simulink model "simplificado"  (R2016a)
settings: Solver=VariableStepAuto  StartTime=0.0  StopTime=10.0  RelTol=1e-3
undefined symbols (not defined in the file or in its folder): h, K1, K2, Kd, Ki, Kp, m, P, pm
libraries: simulink x1
settings Model: Creator=rafael  LastModifiedBy=rafael

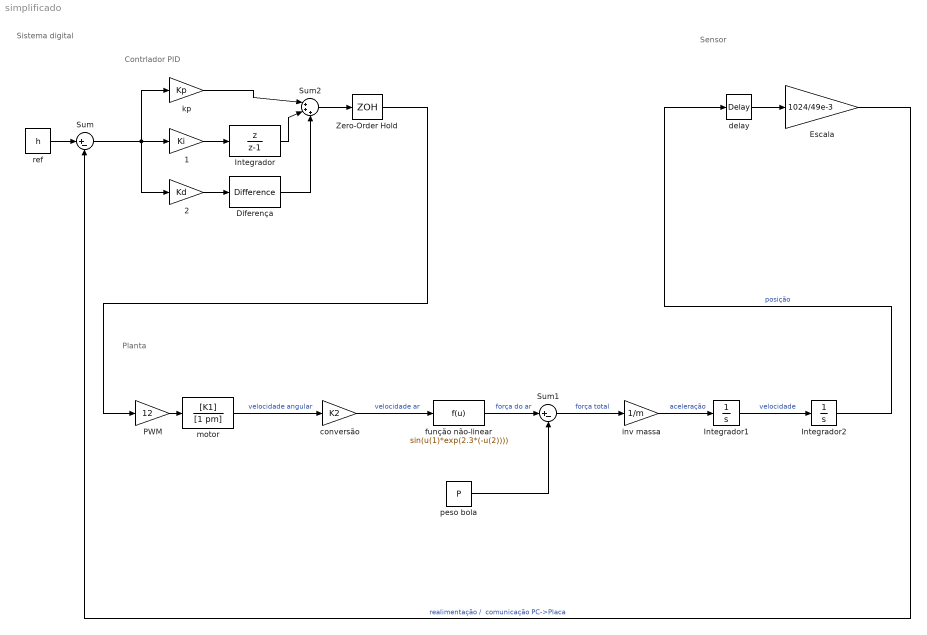
== system simplificado ==
  note: Sistema digital
  note: Sensor
  note: Planta
  note: Contrlador PID
  " 1" : Gain  Gain=Ki
  " 2" : Gain  Gain=Kd
  " motor" : TransferFcn  Numerator=[K1]  Denominator=[1 pm]
  Diferença : simulink/Discrete/Difference  ICPrevInput=0.0  OutMin=[]  OutMax=[]  OutDataType=fixdt(1, 16)  OutScaling=2^-10  DoSatur=off
  Escala : Gain  Gain=1024/49e-3
  "Integrador " : DiscreteTransferFcn  Numerator=[1 0]  Denominator=[1 -1]
  Integrador1 : Integrator
  Integrador2 : Integrator
  PWM : Gain  Gain=12
  Sum : Sum  Inputs=|+-
  Sum1 : Sum  Inputs=|+-
  Sum2 : Sum  Inputs=|+++
  Zero-Order Hold : ZeroOrderHold
  conversão : Gain  Gain=K2
  delay : TransportDelay
  função não-linear : Fcn  Expr=sin(u(1)*exp(2.3*(-u(2))))
  inv massa : Gain  Gain=1/m
  "kp " : Gain  Gain=Kp
  peso bola : Constant  Value=P
  ref : Constant  Value=h
  wires:
  ref/1 -> Sum/1
  " motor"/1 -> conversão/1  "velocidade angular"
  conversão/1 -> função não-linear/1  "velocidade ar"
  função não-linear/1 -> Sum1/1  "força do ar"
  peso bola/1 -> Sum1/2
  Sum1/1 -> inv massa/1  "força total"
  inv massa/1 -> Integrador1/1  "aceleração"
  Integrador1/1 -> Integrador2/1  "velocidade"
  PWM/1 -> " motor"/1
  delay/1 -> Escala/1
  Zero-Order Hold/1 -> PWM/1
  " 1"/1 -> "Integrador "/1
  " 2"/1 -> Diferença/1
  "kp "/1 -> Sum2/1
  "Integrador "/1 -> Sum2/2
  Diferença/1 -> Sum2/3
  Sum2/1 -> Zero-Order Hold/1
  Sum/1 -> "kp "/1, " 2"/1, " 1"/1
  Integrador2/1 -> delay/1  "posição"
  Escala/1 -> Sum/2  "realimentação /  comunicação PC->Placa"
